simulink model "robot_lqr_model"  (R2024b)
settings: Solver=VariableStepAuto  StartTime=0.0  StopTime=10.0  RelTol=1e-3
model workspace (MAT data in the model file):
  pitchd = Simulink.Parameter
  pitchd.Value = 1
  pitchd.Complexity = 'real'
  pitchd.Dimensions = [1 1]
  pitchd.DataType = 'auto'
  yawd = Simulink.Parameter
  yawd.Value = 1
  yawd.Complexity = 'real'
  yawd.Dimensions = [1 1]
  yawd.DataType = 'auto'
values from neighbouring files (symbols this model uses):
  A = [0   1.0000        0        0 ... (first row only)    [invgui.m]    (also in p1.m = 14; p2.m = 14; robot.m = [0 1 0 0; robot_cascade.m = [ 0, 1, 0, 0)
  B = [0; 1.8182; 0; 4.5455]    [invgui.m]    (also in p1.m = 18; p2.m = 18; robot.m = B ./ R; robot_cascade.m = B ./ r_wheel)
  C_xt = eye(4)    [robot.m]    (also in robot_cascade.m; robot_linear.m; robot_lqr.m)
  D_xt = [0;0;0;0]    [robot.m]    (also in robot_cascade.m; robot_linear.m; robot_lqr.m)
  K = plot([cartpos(1) pendx(1)], [0.03 pendy(1)], 'b',     'LineWidth',[7])    [invgui.m]    (also in robot_lqr.m = lqr(A,B,Q,R))
  Km = 0.212207    [robot.m]    (also in robot_cascade.m = 16.1290322581; robot_linear.m; robot_lqr.m)
  n = 18.75    [robot.m]    (also in robot_cascade.m; robot_linear.m; robot_lqr.m)
libraries: cstblocks x10
settings Model: Creator=cosr3  LastModifiedBy=cosr3

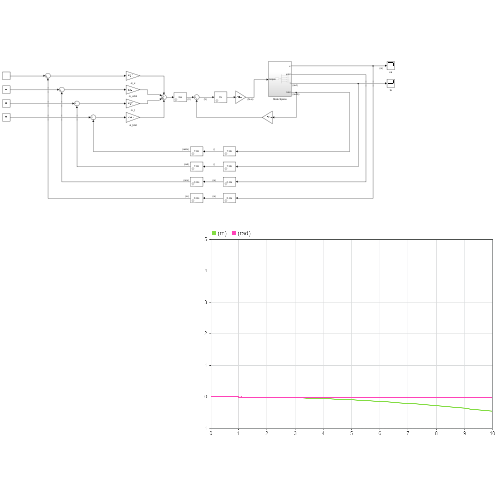
[thumbnail: Simulink's stored preview of the top-level diagram]
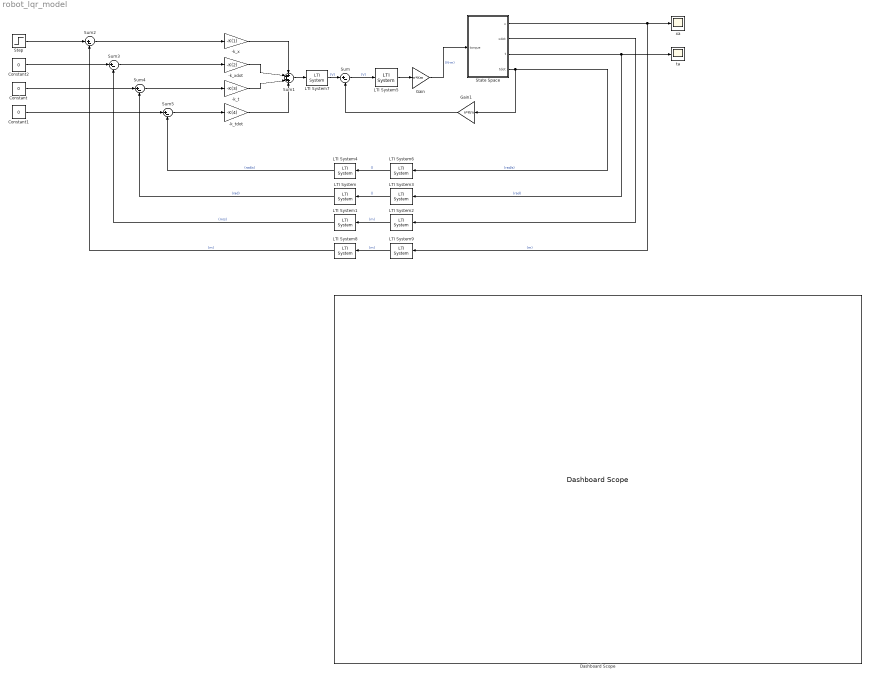
== system robot_lqr_model ==
  -k_t : Gain  Gain=-K(3)
  -k_tdot : Gain  Gain=-K(4)
  -k_x : Gain  Gain=-K(1)
  -k_xdot : Gain  Gain=-K(2)
  Constant : Constant  Value=0
  Constant1 : Constant  Value=0
  Constant2 : Constant  Value=0
  Dashboard Scope : DashboardScope  TimeSpan=10  Ymin=-1  Ymax=5  ScaleAtStop=off
  Gain : Gain  Gain=n*Km
  Gain1 : Gain  Gain=n*Km
  LTI System : cstblocks/LTI System  sys=T.Hc  IC=[]  PadeOrder=0
  LTI System1 : cstblocks/LTI System  sys=X.Hc  IC=[]  PadeOrder=0
  LTI System2 : cstblocks/LTI System  sys=X.Hs  IC=[]  PadeOrder=0
  LTI System3 : cstblocks/LTI System  sys=T.Hs  IC=[]  PadeOrder=0
  LTI System4 : cstblocks/LTI System  sys=T.Hc  IC=[]  PadeOrder=0
  LTI System5 : cstblocks/LTI System  sys=Ye  IC=[]  PadeOrder=0
  LTI System6 : cstblocks/LTI System  sys=T.Hs  IC=[]  PadeOrder=0
  LTI System7 : cstblocks/LTI System  sys=Ga  IC=[]  PadeOrder=0
  LTI System8 : cstblocks/LTI System  sys=X.Hc  IC=[]  PadeOrder=0
  LTI System9 : cstblocks/LTI System  sys=X.Hs  IC=[]  PadeOrder=0
  State Space : Subsystem
  Step : Step  SampleTime=0
  Sum{,2..5} (5 alike) : Sum  Inputs=|+-
  Sum1 : Sum  Inputs=++++
  ta : Scope
  xa : Scope
  wires:
  LTI System5/1 -> Gain/1
  Gain/1 -> State Space/1(torque)  "(N-m)"
  LTI System3/1 -> LTI System/1  "()"
  LTI System2/1 -> LTI System1/1  "(m)"
  Sum/1 -> LTI System5/1  "(V)"
  Gain1/1 -> Sum/2
  LTI System7/1 -> Sum/1  "(V)"
  State Space/1(x) -> LTI System9/1, xa/1  "(m)"
  State Space/4(tdot) -> Gain1/1, LTI System6/1  "(rad/s)"
  State Space/3(t) -> LTI System3/1, ta/1  "(rad)"
  LTI System6/1 -> LTI System4/1  "()"
  LTI System9/1 -> LTI System8/1  "(m)"
  State Space/2(xdot) -> LTI System2/1
  Sum1/1 -> LTI System7/1
  -k_x/1 -> Sum1/1
  -k_xdot/1 -> Sum1/2
  -k_t/1 -> Sum1/3
  -k_tdot/1 -> Sum1/4
  Sum2/1 -> -k_x/1
  Sum3/1 -> -k_xdot/1
  Sum4/1 -> -k_t/1
  Sum5/1 -> -k_tdot/1
  Step/1 -> Sum2/1
  Constant2/1 -> Sum3/1
  Constant/1 -> Sum4/1
  Constant1/1 -> Sum5/1
  LTI System4/1 -> Sum5/2  "(rad/s)"
  LTI System/1 -> Sum4/2  "(rad)"
  LTI System1/1 -> Sum3/2  "(m/s)"
  LTI System8/1 -> Sum2/2  "(m)"

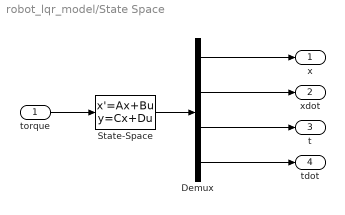
== system robot_lqr_model/State Space ==
  torque : Inport
  Demux : Demux
  State-Space : StateSpace  A=A  B=B  C=C_xt  D=D_xt  InitialCondition=0
  x : Outport
  xdot : Outport  Port=2
  t : Outport  Port=3
  tdot : Outport  Port=4
  wires:
  Demux/1 -> x/1
  State-Space/1 -> Demux/1
  Demux/4 -> tdot/1
  Demux/2 -> xdot/1
  torque/1 -> State-Space/1
  Demux/3 -> t/1
